simulink model "rp_modelling_nl"  (R2023b)
settings: Solver=VariableStepAuto  StartTime=0.0  StopTime=10.0  RelTol=1e-6  AbsTol=1e-6
values from neighbouring files (symbols this model uses):
  rp_p = rp_parameters()    [rp_mainfile_modelling_comparison_a.m]    (also in rp_mainfile_modelling_comparison_b.m)
undefined symbols (not defined in the file or in its folder): rp_nl_model
settings Model: Creator=gory  LastModifiedBy=cgorman

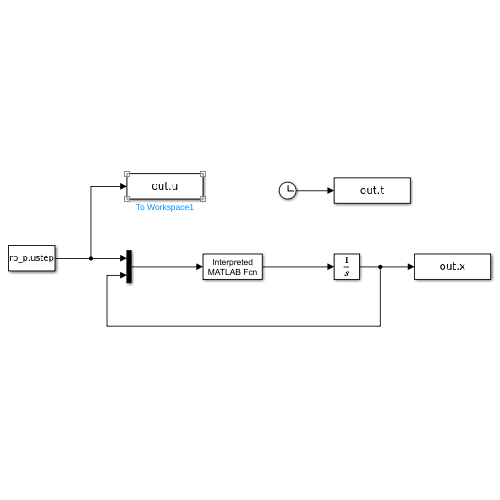
[thumbnail: Simulink's stored preview of the top-level diagram]
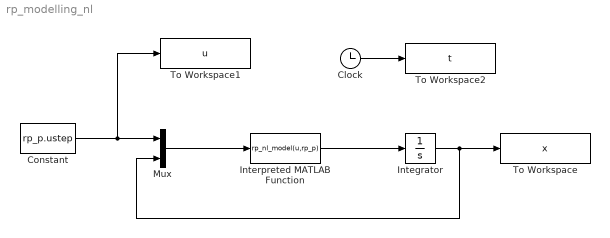
== system rp_modelling_nl ==
  Clock : Clock
  Constant : Constant  Value=rp_p.ustep
  Integrator : Integrator  InitialCondition=rp_p.ic
  Interpreted MATLAB Function : MATLABFcn  MATLABFcn=rp_nl_model(u,rp_p)
  Mux : Mux  Inputs=2
  To Workspace : ToWorkspace  VariableName=x  SampleTime=-1
  To Workspace1 : ToWorkspace  VariableName=u  SampleTime=-1
  To Workspace2 : ToWorkspace  VariableName=t  SampleTime=-1
  wires:
  Mux/1 -> Interpreted MATLAB Function/1
  Interpreted MATLAB Function/1 -> Integrator/1
  Constant/1 -> To Workspace1/1, Mux/1
  Integrator/1 -> To Workspace/1, Mux/2
  Clock/1 -> To Workspace2/1
